simulink model "BatchTest_2024"  (R2023b)
settings: Solver=FixedStepDiscrete  StartTime=0.0  StopTime=100  FixedStep=0.001  RelTol=1e-3  EnableMultiTasking=on
PostLoadFcn:
  | , if any(exist('dsrtsu_mdlpostloadfcn', 'file') == [2, 3, 6]), try dsrtsu_mdlpostloadfcn('Execute', bdroot); catch fprintf('Error in PostLoadFcn (dsrtsu_mdlpostloadfcn) for model "%s":\n %s\n', bdroot, lasterr); end, end,
libraries: simulink x2
settings Model: DSRTSU_INTERNAL_RTI_VER=460  DSRTSU_INTERNAL_RTI_TYPE=rti1401  DSRTSU_INTERNAL_RTIFPGA=50  Creator=jreuter  LastModifiedBy=jreuter
settings SolverCC: AlgebraicLoopSolver=TrustRegion
settings DataIOCC: SaveFormat=Array  ReturnWorkspaceOutputs=off
settings OptimizationCC: BlockReduction=off  OptimizeBlockIOStorage=off  BufferReuse=off  GlobalBufferReuse=off  ExpressionFolding=off  LocalBlockOutputs=off  LifeSpan=inf
settings DebuggingCC: UnconnectedInputMsg=warning  UnconnectedOutputMsg=warning  UnconnectedLineMsg=warning  SFUnexpectedBacktrackingDiag=warning  SFNoUnconditionalDefaultTransitionDiag=warning  SFExecutionAtInitializationDiag=none  ArithmeticOperatorsInVariantConditions=warning
settings HardwareCC: ProdBitPerPointer=32  ProdBitPerSizeT=32  ProdBitPerPtrDiffT=32  ProdLargestAtomicFloat=None  ProdEndianess=BigEndian  ProdWordSize=32  ProdHWDeviceType=Generic->Custom  TargetIntDivRoundTo=Zero  TargetEndianess=BigEndian  TargetHWDeviceType=Generic->Custom
settings ModelReferenceCC: EnableRefExpFcnMdlSchedulingChecks=on  PropagateSignalLabelsOutOfModel=off
settings SFSimCC: SimUseLocalCustomCode=off  CustomCodeUndefinedFunction=UseInterfaceOnly
settings RTWCC: Description=dSPACE DS1104 Hardware Platform  SystemTargetFile=rti1104.tlc  MakeCommand=make_rti  TemplateMakefile=rti1104.tmf  RTWUseLocalCustomCode=off  DLArmComputeVersion=19.05
settings CodeAppCC: StateflowObjectComments=on
settings STFCustomTargetCC: TargetLangStandard=C89/C90 (ANSI)  ParMdlRefBuildCompliant=on  MatFileLogging=on  GRTInterface=on  SystemTargetFile=rti1104.tlc
settings GRTTargetCC: TargetLangStandard=C89/C90 (ANSI)  CompOptLevelCompliant=off  ConcurrentExecutionCompliant=off  CombineOutputUpdateFcns=off  CPPClassGenCompliant=off  GRTInterface=on  UseToolchainInfoCompliant=off  ExtModeMexFile=noextcomm
settings ConfigComp: CovMetricSettings=dw  CovSaveCumulativeToWorkspaceVar=on  CovSaveSingleToWorkspaceVar=on  CovExternalEMLEnable=off

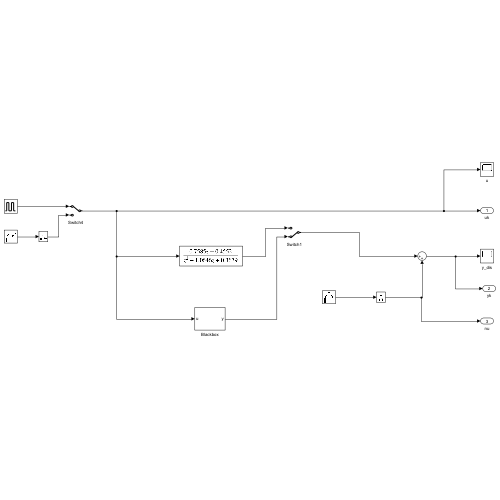
[thumbnail: Simulink's stored preview of the top-level diagram]
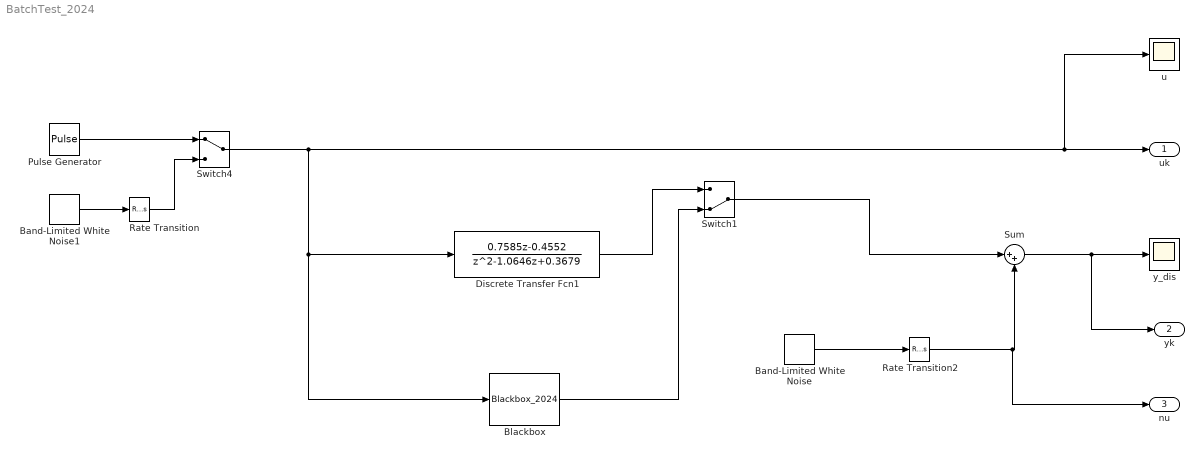
== system BatchTest_2024 ==
  Band-Limited White Noise : simulink/Sources/Band-Limited White Noise  Cov=1e-9  Ts=.1  seed=[23341]
  Band-Limited White Noise1 : simulink/Sources/Band-Limited White Noise  Cov=4  Ts=.1  seed=[23341]
  Blackbox : S-Function  FunctionName=Blackbox_2024  SFunctionDeploymentMode=off  EnableBusSupport=off
      mask Display:
      | port_label('input',1,'u')
      | port_label('output',1,'y')
  Discrete Transfer Fcn1 : DiscreteTransferFcn  Numerator=[0.7585 -0.4552]  Denominator=[1 -1.0646 0.3679]
  Pulse Generator : DiscretePulseGenerator  PulseType=Time based  Amplitude=20  Period=1  PulseWidth=50
  Rate Transition : RateTransition  Integrity=off  OutPortSampleTimeOpt=Inherit
  Rate Transition2 : RateTransition  Integrity=off  OutPortSampleTimeOpt=Inherit
  Sum : Sum  Inputs=|++
  Switch1 : ManualSwitch  CurrentSetting=0
  Switch4 : ManualSwitch
  u : Scope
  y_dis : Scope
  uk : Outport
  yk : Outport  Port=2
  nu : Outport  Port=3
  wires:
  Band-Limited White Noise1/1 -> Rate Transition/1
  Band-Limited White Noise/1 -> Rate Transition2/1
  Pulse Generator/1 -> Switch4/1
  Rate Transition/1 -> Switch4/2
  Rate Transition2/1 -> Sum/2, nu/1
  Sum/1 -> yk/1, y_dis/1
  Switch4/1 -> Discrete Transfer Fcn1/1, Blackbox/1, u/1, uk/1
  Discrete Transfer Fcn1/1 -> Switch1/1
  Blackbox/1 -> Switch1/2
  Switch1/1 -> Sum/1
